simulink model "gm_inc_enc_v26_vnl"  (R2022b)
settings: Solver=FixedStepDiscrete  StartTime=0.0  StopTime=SimulationsDauer  RelTol=1e-3
undefined symbols (not defined in the file or in its folder): CW_CCW_Switch, d_axis_hit_CompareValue, DiscIntNeverNeededParam, f_ISR, IncPerTurn, inital_zero_speed_timeout, n_max, Offset_Position_elec, Offset_Position_mech, OmegaPerOverSampl, Periode, Phase_Delay_A, Phase_Delay_B, PolePair, QuadratureFactor, reciprocal_iterations, T_fpga, T_mech
libraries: simulink x25, hdlsllib x11, hdlmdlgenlib x4, dspsrcs4 x3, dspswit3 x2, spsEdgeDetectorLib x2, simulink_extras x1
(part 1 of 5)
settings Model: Creator=Wendel_ELSYS  LastModifiedBy=Admin
settings SolverCC: ConcurrentTasks=on  AlgebraicLoopSolver=TrustRegion  MinimalZcImpactIntegration=on
settings DataIOCC: LimitDataPoints=on  SaveFormat=Array
settings OptimizationCC: BlockReduction=off  ConditionallyExecuteInputs=off  DefaultParameterBehavior=Inlined  InheritOutputTypeSmallerThanSingle=on  LifeSpan=inf
settings DebuggingCC: ReadBeforeWriteMsg=DisableAll  WriteAfterWriteMsg=DisableAll  WriteAfterReadMsg=DisableAll  AlgebraicLoopMsg=error  InheritedTsInSrcMsg=none  SingleTaskRateTransMsg=error  ParameterOverflowMsg=none  UnconnectedInputMsg=warning  UnconnectedOutputMsg=warning  UnconnectedLineMsg=warning  SFUnexpectedBacktrackingDiag=warning  SFNoUnconditionalDefaultTransitionDiag=warning  SFExecutionAtInitializationDiag=none  SFMachineParentedDataDiag=warning  ArithmeticOperatorsInVariantConditions=warning
settings HardwareCC: ProdBitPerPointer=32  ProdBitPerSizeT=32  ProdBitPerPtrDiffT=32  ProdLargestAtomicFloat=None  ProdIntDivRoundTo=Undefined  ProdEndianess=Unspecified  ProdWordSize=32  ProdHWDeviceType=ASIC/FPGA->ASIC/FPGA  ProdEqTarget=off
settings ModelReferenceCC: UpdateModelReferenceTargets=IfOutOfDate  EnableRefExpFcnMdlSchedulingChecks=on  PropagateSignalLabelsOutOfModel=off
settings SFSimCC: SFSimEcho=off  SimUseLocalCustomCode=off  CustomCodeUndefinedFunction=UseInterfaceOnly
settings RTWCC: RTWUseLocalCustomCode=off  DLArmComputeVersion=19.05
settings CodeAppCC: StateflowObjectComments=on
settings GRTTargetCC: TargetLangStandard=C89/C90 (ANSI)
settings ConfigComp: CovMetricSettings=dw  CovSaveCumulativeToWorkspaceVar=on  CovSaveSingleToWorkspaceVar=on  CovExternalEMLEnable=off
settings SimscapeCC: SimscapeNormalizeSystem=off

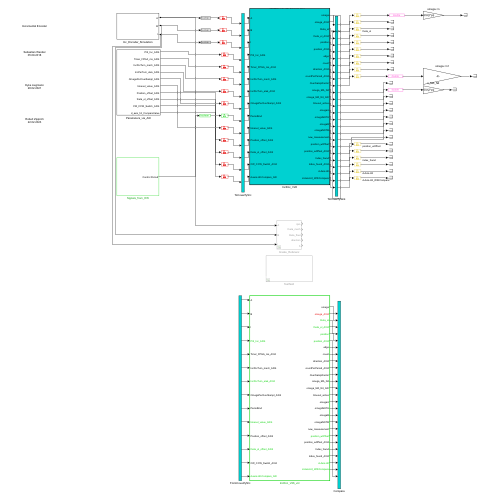
[thumbnail: Simulink's stored preview of the top-level diagram]
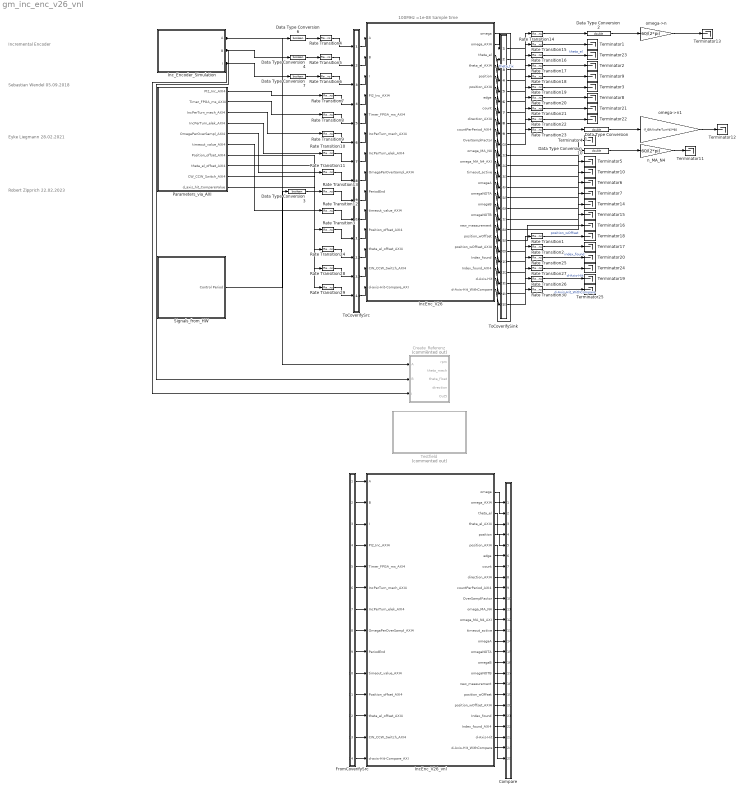
== system gm_inc_enc_v26_vnl ==
  note: 100MHz =1e-08 Sample time
  note: Sebastian Wendel
      | 05.09.2018
  note: Incremental Encoder
  note: Eyke Liegmann
      | 28.02.2021
  note: Robert Zipprich
      | 22.02.2023
  Compare : Subsystem
      mask Display: disp('')
  Create_Referenz : Subsystem  Commented=on
  Data Type Conversion1 : DataTypeConversion  OutDataTypeStr=double  SaturateOnIntegerOverflow=off  RndMeth=Floor
  Data Type Conversion10 : DataTypeConversion  OutDataTypeStr=double  SaturateOnIntegerOverflow=off  RndMeth=Floor
  Data Type Conversion2 : DataTypeConversion  OutDataTypeStr=double  SaturateOnIntegerOverflow=off  RndMeth=Floor
  Data Type Conversion{3..4,6..7} (4 alike) : DataTypeConversion  OutDataTypeStr=boolean  SaturateOnIntegerOverflow=off  RndMeth=Floor
  FromCoverifySrc : Subsystem
      mask Display: disp('')
  IncEnc_V26 : Subsystem  TreatAsAtomicUnit=on
  IncEnc_V26_vnl : Subsystem  TreatAsAtomicUnit=on
  Inc_Encoder_Simulation : Subsystem
  Parameters_via_AXI : Subsystem
  Rate Transition{1..2,14..23,25..27,30} (16 alike) : RateTransition  Deterministic=off  OutPortSampleTime=T_mech
  Rate Transition{3..13,24,28..29} (14 alike) : RateTransition  Deterministic=off  OutPortSampleTime=T_fpga
  Signals_from_HW : Subsystem
  Terminator{1..25} (25 alike) : Terminator
  Testfield : Subsystem  Commented=on
  ToCoverifySink : Subsystem
      mask Display: disp('')
  ToCoverifySrc : Subsystem
      mask Display: disp('')
  n_MA_N4 : Gain  Gain=60/(2*pi)  OutDataTypeStr=double
  omega->n : Gain  Gain=60/(2*pi)  OutDataTypeStr=double
  omega->n1 : Gain  Gain=(f_ISR/(IncPerTurn*4))*60  OutDataTypeStr=double
  wires:
  Data Type Conversion6/1 -> Rate Transition4/1
  Data Type Conversion4/1 -> Rate Transition5/1
  Data Type Conversion7/1 -> Rate Transition6/1
  omega->n/1 -> Terminator13/1
  Data Type Conversion2/1 -> omega->n/1
  Data Type Conversion1/1 -> omega->n1/1
  Data Type Conversion3/1 -> Rate Transition13/1
  Rate Transition14/1 -> Data Type Conversion2/1
  Rate Transition15/1 -> Terminator1/1
  Rate Transition17/1 -> Terminator2/1
  Rate Transition19/1 -> Terminator3/1
  Rate Transition23/1 -> Data Type Conversion1/1
  Data Type Conversion10/1 -> n_MA_N4/1
  Rate Transition20/1 -> Terminator8/1
  Rate Transition18/1 -> Terminator9/1
  n_MA_N4/1 -> Terminator11/1
  omega->n1/1 -> Terminator12/1
  Parameters_via_AXI/1(PI2_Inc_AXI4) -> Rate Transition7/1
  Parameters_via_AXI/2(Timer_FPGA_ms_AXI4) -> Rate Transition8/1
  Parameters_via_AXI/3(IncPerTurn_mech_AXI4) -> Rate Transition9/1
  Parameters_via_AXI/4(IncPerTurn_elek_AXI4) -> Rate Transition10/1
  Parameters_via_AXI/5(OmegaPerOverSampl_AXI4) -> Rate Transition11/1
  Parameters_via_AXI/6(timeout_value_AXI4) -> Rate Transition12/1
  Inc_Encoder_Simulation/2(B) -> Create_Referenz/2(B), Data Type Conversion4/1
  Inc_Encoder_Simulation/3(I) -> Create_Referenz/3(I), Data Type Conversion7/1
  Inc_Encoder_Simulation/1(A) -> Data Type Conversion6/1, Create_Referenz/1(A)
  Signals_from_HW/1(Control Period) -> Data Type Conversion3/1
  Rate Transition1/1 -> Terminator18/1  "position_wOffset"
  Rate Transition2/1 -> Terminator17/1
  Parameters_via_AXI/7(Position_offset_AXI4) -> Rate Transition3/1
  Parameters_via_AXI/8(theta_el_offset_AXI4) -> Rate Transition24/1
  Rate Transition25/1 -> Terminator20/1  "index_found"
  Rate Transition26/1 -> Terminator19/1  "d-Axis-Hit"
  Rate Transition22/1 -> Terminator22/1
  Rate Transition21/1 -> Terminator21/1
  Rate Transition16/1 -> Terminator23/1  "theta_el"
  Rate Transition27/1 -> Terminator24/1
  Parameters_via_AXI/9(CW_CCW_Switch_AXI4) -> Rate Transition28/1
  Parameters_via_AXI/10(d_axis_hit_CompareValue) -> Rate Transition29/1
  Rate Transition30/1 -> Terminator25/1  "d-Axis-Hit_WithCompare"
  ToCoverifySrc/1(out1) -> IncEnc_V26/1(A)
  ToCoverifySrc/2(out2) -> IncEnc_V26/2(B)
  ToCoverifySrc/3(out3) -> IncEnc_V26/3(I)
  ToCoverifySrc/4(out4) -> IncEnc_V26/4(PI2_Inc_AXI4)
  ToCoverifySrc/5(out5) -> IncEnc_V26/5(Timer_FPGA_ms_AXI4)
  ToCoverifySrc/6(out6) -> IncEnc_V26/6(IncPerTurn_mech_AXI4)
  ToCoverifySrc/7(out7) -> IncEnc_V26/7(IncPerTurn_elek_AXI4)
  ToCoverifySrc/8(out8) -> IncEnc_V26/8(OmegaPerOverSampl_AXI4)
  ToCoverifySrc/9(out9) -> IncEnc_V26/9(PeriodEnd)
  ToCoverifySrc/10(out10) -> IncEnc_V26/10(timeout_value_AXI4)
  ToCoverifySrc/11(out11) -> IncEnc_V26/11(Position_offset_AXI4)
  ToCoverifySrc/12(out12) -> IncEnc_V26/12(theta_el_offset_AXI4)
  ToCoverifySrc/13(out13) -> IncEnc_V26/13(CW_CCW_Switch_AXI4)
  ToCoverifySrc/14(out14) -> IncEnc_V26/14(d-axis-Hit-Compare_AXI)
  IncEnc_V26/1(omega) -> ToCoverifySink/1(in1)
  IncEnc_V26/2(omega_AXI4) -> ToCoverifySink/2(in2)
  IncEnc_V26/3(theta_el) -> ToCoverifySink/3(in3)  "theta_fix"
  IncEnc_V26/4(theta_el_AXI4) -> ToCoverifySink/4(in4)
  IncEnc_V26/5(position) -> ToCoverifySink/5(in5)
  IncEnc_V26/6(position_AXI4) -> ToCoverifySink/6(in6)
  IncEnc_V26/7(edge) -> ToCoverifySink/7(in7)
  IncEnc_V26/8(count) -> ToCoverifySink/8(in8)
  IncEnc_V26/9(direction_AXI4) -> ToCoverifySink/9(in9)
  IncEnc_V26/10(countPerPeriod_AXI4) -> ToCoverifySink/10(in10)
  IncEnc_V26/11(OverSamplFactor) -> ToCoverifySink/11(in11)
  IncEnc_V26/12(omega_MA_N4) -> ToCoverifySink/12(in12)
  IncEnc_V26/13(omega_MA_N4_AXI) -> ToCoverifySink/13(in13)
  IncEnc_V26/14(timeout_active) -> ToCoverifySink/14(in14)
  IncEnc_V26/15(omegaA) -> ToCoverifySink/15(in15)
  IncEnc_V26/16(omegaNOTA) -> ToCoverifySink/16(in16)
  IncEnc_V26/17(omegaB) -> ToCoverifySink/17(in17)
  IncEnc_V26/18(omegaNOTB) -> ToCoverifySink/18(in18)
  IncEnc_V26/19(new_measurement) -> ToCoverifySink/19(in19)
  IncEnc_V26/20(position_wOffset) -> ToCoverifySink/20(in20)
  IncEnc_V26/21(position_wOffset_AXI4) -> ToCoverifySink/21(in21)
  IncEnc_V26/22(Index_found) -> ToCoverifySink/22(in22)
  IncEnc_V26/23(Index_found_AXI4) -> ToCoverifySink/23(in23)
  IncEnc_V26/24(d-Axis-Hit) -> ToCoverifySink/24(in24)
  IncEnc_V26/25(d-Axis-Hit_WithCompare) -> ToCoverifySink/25(in25)
  Rate Transition4/1 -> ToCoverifySrc/1(in1)
  Rate Transition5/1 -> ToCoverifySrc/2(in2)
  Rate Transition6/1 -> ToCoverifySrc/3(in3)
  Rate Transition7/1 -> ToCoverifySrc/4(in4)
  Rate Transition8/1 -> ToCoverifySrc/5(in5)
  Rate Transition9/1 -> ToCoverifySrc/6(in6)
  Rate Transition10/1 -> ToCoverifySrc/7(in7)
  Rate Transition11/1 -> ToCoverifySrc/8(in8)
  Rate Transition13/1 -> ToCoverifySrc/9(in9)
  Rate Transition12/1 -> ToCoverifySrc/10(in10)
  Rate Transition3/1 -> ToCoverifySrc/11(in11)
  Rate Transition24/1 -> ToCoverifySrc/12(in12)
  Rate Transition28/1 -> ToCoverifySrc/13(in13)
  Rate Transition29/1 -> ToCoverifySrc/14(in14)
  ToCoverifySink/1(out1) -> Rate Transition14/1
  ToCoverifySink/2(out2) -> Rate Transition15/1
  ToCoverifySink/3(out3) -> Rate Transition16/1
  ToCoverifySink/4(out4) -> Rate Transition17/1
  ToCoverifySink/5(out5) -> Rate Transition18/1
  ToCoverifySink/6(out6) -> Rate Transition19/1
  ToCoverifySink/7(out7) -> Rate Transition20/1
  ToCoverifySink/8(out8) -> Rate Transition21/1
  ToCoverifySink/9(out9) -> Rate Transition22/1
  ToCoverifySink/10(out10) -> Rate Transition23/1
  ToCoverifySink/11(out11) -> Terminator4/1
  ToCoverifySink/12(out12) -> Data Type Conversion10/1
  ToCoverifySink/13(out13) -> Terminator5/1
  ToCoverifySink/14(out14) -> Terminator10/1
  ToCoverifySink/15(out15) -> Terminator6/1
  ToCoverifySink/16(out16) -> Terminator7/1
  ToCoverifySink/17(out17) -> Terminator14/1
  ToCoverifySink/18(out18) -> Terminator15/1
  ToCoverifySink/19(out19) -> Terminator16/1
  ToCoverifySink/20(out20) -> Rate Transition1/1
  ToCoverifySink/21(out21) -> Rate Transition2/1
  ToCoverifySink/22(out22) -> Rate Transition25/1
  ToCoverifySink/23(out23) -> Rate Transition27/1
  ToCoverifySink/24(out24) -> Rate Transition26/1
  ToCoverifySink/25(out25) -> Rate Transition30/1
  FromCoverifySrc/1(out1) -> IncEnc_V26_vnl/1(A)
  FromCoverifySrc/2(out2) -> IncEnc_V26_vnl/2(B)
  FromCoverifySrc/3(out3) -> IncEnc_V26_vnl/3(I)
  FromCoverifySrc/4(out4) -> IncEnc_V26_vnl/4(PI2_Inc_AXI4)
  FromCoverifySrc/5(out5) -> IncEnc_V26_vnl/5(Timer_FPGA_ms_AXI4)
  FromCoverifySrc/6(out6) -> IncEnc_V26_vnl/6(IncPerTurn_mech_AXI4)
  FromCoverifySrc/7(out7) -> IncEnc_V26_vnl/7(IncPerTurn_elek_AXI4)
  FromCoverifySrc/8(out8) -> IncEnc_V26_vnl/8(OmegaPerOverSampl_AXI4)
  FromCoverifySrc/9(out9) -> IncEnc_V26_vnl/9(PeriodEnd)
  FromCoverifySrc/10(out10) -> IncEnc_V26_vnl/10(timeout_value_AXI4)
  FromCoverifySrc/11(out11) -> IncEnc_V26_vnl/11(Position_offset_AXI4)
  FromCoverifySrc/12(out12) -> IncEnc_V26_vnl/12(theta_el_offset_AXI4)
  FromCoverifySrc/13(out13) -> IncEnc_V26_vnl/13(CW_CCW_Switch_AXI4)
  FromCoverifySrc/14(out14) -> IncEnc_V26_vnl/14(d-axis-Hit-Compare_AXI)
  IncEnc_V26_vnl/1(omega) -> Compare/1(in1)
  IncEnc_V26_vnl/2(omega_AXI4) -> Compare/2(in2)
  IncEnc_V26_vnl/3(theta_el) -> Compare/3(in3)
  IncEnc_V26_vnl/4(theta_el_AXI4) -> Compare/4(in4)
  IncEnc_V26_vnl/5(position) -> Compare/5(in5)
  IncEnc_V26_vnl/6(position_AXI4) -> Compare/6(in6)
  IncEnc_V26_vnl/7(edge) -> Compare/7(in7)
  IncEnc_V26_vnl/8(count) -> Compare/8(in8)
  IncEnc_V26_vnl/9(direction_AXI4) -> Compare/9(in9)
  IncEnc_V26_vnl/10(countPerPeriod_AXI4) -> Compare/10(in10)
  IncEnc_V26_vnl/11(OverSamplFactor) -> Compare/11(in11)
  IncEnc_V26_vnl/12(omega_MA_N4) -> Compare/12(in12)
  IncEnc_V26_vnl/13(omega_MA_N4_AXI) -> Compare/13(in13)
  IncEnc_V26_vnl/14(timeout_active) -> Compare/14(in14)
  IncEnc_V26_vnl/15(omegaA) -> Compare/15(in15)
  IncEnc_V26_vnl/16(omegaNOTA) -> Compare/16(in16)
  IncEnc_V26_vnl/17(omegaB) -> Compare/17(in17)
  IncEnc_V26_vnl/18(omegaNOTB) -> Compare/18(in18)
  IncEnc_V26_vnl/19(new_measurement) -> Compare/19(in19)
  IncEnc_V26_vnl/20(position_wOffset) -> Compare/20(in20)
  IncEnc_V26_vnl/21(position_wOffset_AXI4) -> Compare/21(in21)
  IncEnc_V26_vnl/22(Index_found) -> Compare/22(in22)
  IncEnc_V26_vnl/23(Index_found_AXI4) -> Compare/23(in23)
  IncEnc_V26_vnl/24(d-Axis-Hit) -> Compare/24(in24)
  IncEnc_V26_vnl/25(d-Axis-Hit_WithCompare) -> Compare/25(in25)

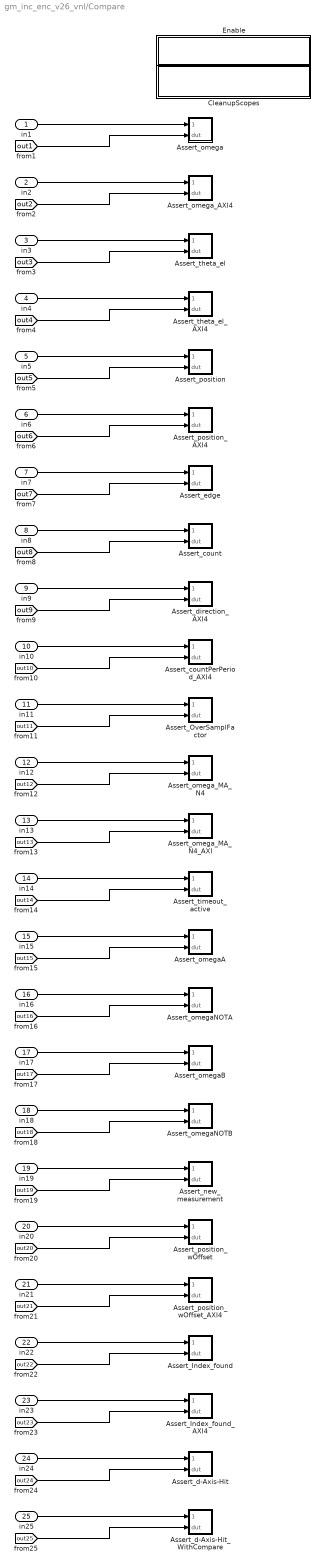
== system gm_inc_enc_v26_vnl/Compare ==
  in1 : Inport
  in2 : Inport  Port=2
  in3 : Inport  Port=3
  in4 : Inport  Port=4
  in5 : Inport  Port=5
  in6 : Inport  Port=6
  in7 : Inport  Port=7
  in8 : Inport  Port=8
  in9 : Inport  Port=9
  in10 : Inport  Port=10
  in11 : Inport  Port=11
  in12 : Inport  Port=12
  in13 : Inport  Port=13
  in14 : Inport  Port=14
  in15 : Inport  Port=15
  in16 : Inport  Port=16
  in17 : Inport  Port=17
  in18 : Inport  Port=18
  in19 : Inport  Port=19
  in20 : Inport  Port=20
  in21 : Inport  Port=21
  in22 : Inport  Port=22
  in23 : Inport  Port=23
  in24 : Inport  Port=24
  in25 : Inport  Port=25
  Assert_Index_found : Subsystem
      settings: LibrarySourceBlock=hdlmdlgenlib/AssertEq
  Assert_Index_found_AXI4 : Subsystem
      settings: LibrarySourceBlock=hdlmdlgenlib/AssertEq
  Assert_OverSamplFactor : Subsystem
      settings: LibrarySourceBlock=hdlmdlgenlib/AssertEq
  Assert_count : Subsystem
      settings: LibrarySourceBlock=hdlmdlgenlib/AssertEq
  Assert_countPerPeriod_AXI4 : Subsystem
      settings: LibrarySourceBlock=hdlmdlgenlib/AssertEq
  Assert_d-Axis-Hit : Subsystem
      settings: LibrarySourceBlock=hdlmdlgenlib/AssertEq
  Assert_d-Axis-Hit_WithCompare : Subsystem
      settings: LibrarySourceBlock=hdlmdlgenlib/AssertEq
  Assert_direction_AXI4 : Subsystem
      settings: LibrarySourceBlock=hdlmdlgenlib/AssertEq
  Assert_edge : Subsystem
      settings: LibrarySourceBlock=hdlmdlgenlib/AssertEq
  Assert_new_measurement : Subsystem
      settings: LibrarySourceBlock=hdlmdlgenlib/AssertEq
  Assert_omega : Subsystem
      settings: LibrarySourceBlock=hdlmdlgenlib/AssertEq
  Assert_omegaA : Subsystem
      settings: LibrarySourceBlock=hdlmdlgenlib/AssertEq
  Assert_omegaB : Subsystem
      settings: LibrarySourceBlock=hdlmdlgenlib/AssertEq
  Assert_omegaNOTA : Subsystem
      settings: LibrarySourceBlock=hdlmdlgenlib/AssertEq
  Assert_omegaNOTB : Subsystem
      settings: LibrarySourceBlock=hdlmdlgenlib/AssertEq
  Assert_omega_AXI4 : Subsystem
      settings: LibrarySourceBlock=hdlmdlgenlib/AssertEq
  Assert_omega_MA_N4 : Subsystem
      settings: LibrarySourceBlock=hdlmdlgenlib/AssertEq
  Assert_omega_MA_N4_AXI : Subsystem
      settings: LibrarySourceBlock=hdlmdlgenlib/AssertEq
  Assert_position : Subsystem
      settings: LibrarySourceBlock=hdlmdlgenlib/AssertEq
  Assert_position_AXI4 : Subsystem
      settings: LibrarySourceBlock=hdlmdlgenlib/AssertEq
  Assert_position_wOffset : Subsystem
      settings: LibrarySourceBlock=hdlmdlgenlib/AssertEq
  Assert_position_wOffset_AXI4 : Subsystem
      settings: LibrarySourceBlock=hdlmdlgenlib/AssertEq
  Assert_theta_el : Subsystem
      settings: LibrarySourceBlock=hdlmdlgenlib/AssertEq
  Assert_theta_el_AXI4 : Subsystem
      settings: LibrarySourceBlock=hdlmdlgenlib/AssertEq
  Assert_timeout_active : Subsystem
      settings: LibrarySourceBlock=hdlmdlgenlib/AssertEq
  CleanupScopes : Subsystem
      settings: OpenFcn=|
      | blkName = gcb; %self block
      | idx = regexp(blkName, '/CleanupScopes$', 'once');
      | blkParent = blkName(1:idx-1);
      | blks=find_system(blkParent, 'LookUnderMasks', 'all','blocktype', 'Scope');
      | for itr = 1:length(blks)
      | 	 hScopeCfg = get_param(blks{itr},'ScopeConfiguration');
      | 	 hScopeCfg.Visible = ~ hScopeCfg.Visible;
      | end
      | drawnow;
      mask Display: fprintf(message('hdlcoder:cosim:vnl_dblclick').getString());
  Enable : Subsystem
      settings: OpenFcn=|
      | blkName = gcb;
      | idx = regexp(blkName, '/Enable$', 'once');
      | blkParent = blkName(1:idx-1);
      | blks=find_system(blkParent, 'LookUnderMasks', 'all','blocktype', 'Assertion');
      | e = get_param(blks{1}, 'Enabled');
      | if strcmp(e, 'on'), f= 'off';, else, f = 'on';, end
      | for ii=1:length(blks), set_param(blks{ii}, 'Enabled', f);, end
      | set_param(gcb, 'MaskDisplay',['fprintf(message(''hdlcoder:cosim:vnl_dblclick_assertions'',','''',upper(e),'''',').getString())']);
      mask Display: fprintf(message('hdlcoder:cosim:vnl_dblclick_assertions','OFF').getString());
  wires:
  in1/1 -> Assert_omega/1(cosim)
  [out1] -> Assert_omega/2(dut)
  in2/1 -> Assert_omega_AXI4/1(cosim)
  [out2] -> Assert_omega_AXI4/2(dut)
  in3/1 -> Assert_theta_el/1(cosim)
  [out3] -> Assert_theta_el/2(dut)
  in4/1 -> Assert_theta_el_AXI4/1(cosim)
  [out4] -> Assert_theta_el_AXI4/2(dut)
  in5/1 -> Assert_position/1(cosim)
  [out5] -> Assert_position/2(dut)
  in6/1 -> Assert_position_AXI4/1(cosim)
  [out6] -> Assert_position_AXI4/2(dut)
  in7/1 -> Assert_edge/1(cosim)
  [out7] -> Assert_edge/2(dut)
  in8/1 -> Assert_count/1(cosim)
  [out8] -> Assert_count/2(dut)
  in9/1 -> Assert_direction_AXI4/1(cosim)
  [out9] -> Assert_direction_AXI4/2(dut)
  in10/1 -> Assert_countPerPeriod_AXI4/1(cosim)
  [out10] -> Assert_countPerPeriod_AXI4/2(dut)
  in11/1 -> Assert_OverSamplFactor/1(cosim)
  [out11] -> Assert_OverSamplFactor/2(dut)
  in12/1 -> Assert_omega_MA_N4/1(cosim)
  [out12] -> Assert_omega_MA_N4/2(dut)
  in13/1 -> Assert_omega_MA_N4_AXI/1(cosim)
  [out13] -> Assert_omega_MA_N4_AXI/2(dut)
  in14/1 -> Assert_timeout_active/1(cosim)
  [out14] -> Assert_timeout_active/2(dut)
  in15/1 -> Assert_omegaA/1(cosim)
  [out15] -> Assert_omegaA/2(dut)
  in16/1 -> Assert_omegaNOTA/1(cosim)
  [out16] -> Assert_omegaNOTA/2(dut)
  in17/1 -> Assert_omegaB/1(cosim)
  [out17] -> Assert_omegaB/2(dut)
  in18/1 -> Assert_omegaNOTB/1(cosim)
  [out18] -> Assert_omegaNOTB/2(dut)
  in19/1 -> Assert_new_measurement/1(cosim)
  [out19] -> Assert_new_measurement/2(dut)
  in20/1 -> Assert_position_wOffset/1(cosim)
  [out20] -> Assert_position_wOffset/2(dut)
  in21/1 -> Assert_position_wOffset_AXI4/1(cosim)
  [out21] -> Assert_position_wOffset_AXI4/2(dut)
  in22/1 -> Assert_Index_found/1(cosim)
  [out22] -> Assert_Index_found/2(dut)
  in23/1 -> Assert_Index_found_AXI4/1(cosim)
  [out23] -> Assert_Index_found_AXI4/2(dut)
  in24/1 -> Assert_d-Axis-Hit/1(cosim)
  [out24] -> Assert_d-Axis-Hit/2(dut)
  in25/1 -> Assert_d-Axis-Hit_WithCompare/1(cosim)
  [out25] -> Assert_d-Axis-Hit_WithCompare/2(dut)

== system gm_inc_enc_v26_vnl/Create_Referenz ==
  note: Überprüfen der Ausgabe:
      | (1/((Wert in Periodfelt von Counter)*Inkremente))*60
      | z.B. (1/((2.5*0.000001)*5000))*60
  A : Inport
  B : Inport  Port=2
  I : Inport  Port=3
  HardwareTimer_FPGA_in_ms*InCrements1 : Constant  Value=T_mech*IncPerTurn  OutDataTypeStr=double  SampleTime=T_mech
  IncrementalEncoder_Floating : Subsystem  Commented=on
  "daQuadraturEncoder " : Gain  Commented=on  Gain=4
  n_aus_theta : Subsystem  Commented=on  TreatAsAtomicUnit=on
  poles : Constant  Value=PolePair  OutDataTypeStr=uint8  SampleTime=T_mech
  rpm : Outport
  theta_mech : Outport  Port=2
  theta_float : Outport  Port=3
  direction : Outport  Port=4
  Out5 : Outport  Port=5
  wires:
  n_aus_theta/1(rpm) -> "daQuadraturEncoder "/1
  A/1 -> IncrementalEncoder_Floating/1(A), n_aus_theta/1(count)
  B/1 -> IncrementalEncoder_Floating/2(B)
  IncrementalEncoder_Floating/3(theta_elec) -> theta_float/1  "theta_float"
  poles/1 -> IncrementalEncoder_Floating/4(poles)
  I/1 -> IncrementalEncoder_Floating/3(I)
  HardwareTimer_FPGA_in_ms*InCrements1/1 -> n_aus_theta/2(T)
  IncrementalEncoder_Floating/4(direction) -> direction/1
  IncrementalEncoder_Floating/1(rpm) -> rpm/1
  "daQuadraturEncoder "/1 -> Out5/1
  IncrementalEncoder_Floating/2(theta_mech) -> theta_mech/1

== system gm_inc_enc_v26_vnl/FromCoverifySrc ==
  out1 : Outport
  out2 : Outport  Port=2
  out3 : Outport  Port=3
  out4 : Outport  Port=4
  out5 : Outport  Port=5
  out6 : Outport  Port=6
  out7 : Outport  Port=7
  out8 : Outport  Port=8
  out9 : Outport  Port=9
  out10 : Outport  Port=10
  out11 : Outport  Port=11
  out12 : Outport  Port=12
  out13 : Outport  Port=13
  out14 : Outport  Port=14
  wires:
  [in1] -> out1/1
  [in2] -> out2/1
  [in3] -> out3/1
  [in4] -> out4/1
  [in5] -> out5/1
  [in6] -> out6/1
  [in7] -> out7/1
  [in8] -> out8/1
  [in9] -> out9/1
  [in10] -> out10/1
  [in11] -> out11/1
  [in12] -> out12/1
  [in13] -> out13/1
  [in14] -> out14/1

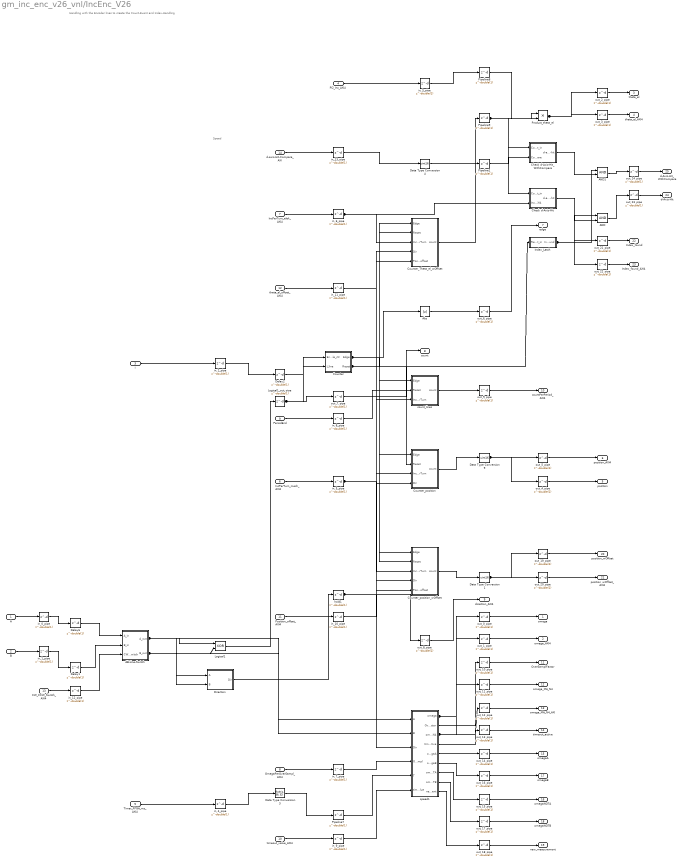
== system gm_inc_enc_v26_vnl/IncEnc_V26 ==
  note: Handling with the Encoder lines to create the Count-Event and Index-Handling
  note: Speed
  A : Inport  OutDataTypeStr=boolean  PortDimensions=1  SampleTime=1e-08
  B : Inport  Port=2  OutDataTypeStr=boolean  PortDimensions=1  SampleTime=1e-08
  I : Inport  Port=3  OutDataTypeStr=boolean  PortDimensions=1  SampleTime=1e-08
  PI2_Inc_AXI4 : Inport  Port=4  OutDataTypeStr=fixdt(0, 24, 24)  PortDimensions=1  SampleTime=1e-08
  Timer_FPGA_ms_AXI4 : Inport  Port=5  OutDataTypeStr=fixdt(0, 32, 32)  PortDimensions=1  SampleTime=1e-08
  IncPerTurn_mech_AXI4 : Inport  Port=6  OutDataTypeStr=uint16  PortDimensions=1  SampleTime=1e-08
  IncPerTurn_elek_AXI4 : Inport  Port=7  OutDataTypeStr=uint16  PortDimensions=1  SampleTime=1e-08
  OmegaPerOverSampl_AXI4 : Inport  Port=8  OutDataTypeStr=fixdt(1, 24, 11)  PortDimensions=1  SampleTime=1e-08
  PeriodEnd : Inport  Port=9  OutDataTypeStr=boolean  PortDimensions=1  SampleTime=1e-08
  timeout_value_AXI4 : Inport  Port=10  OutDataTypeStr=uint32  PortDimensions=1  SampleTime=1e-08
  Position_offset_AXI4 : Inport  Port=11  OutDataTypeStr=uint16  PortDimensions=1  SampleTime=1e-08
  theta_el_offset_AXI4 : Inport  Port=12  OutDataTypeStr=uint16  PortDimensions=1  SampleTime=1e-08
  CW_CCW_Switch_AXI4 : Inport  Port=13  OutDataTypeStr=boolean  PortDimensions=1  SampleTime=1e-08
  d-axis-Hit-Compare_AXI : Inport  Port=14  OutDataTypeStr=uint32  PortDimensions=1  SampleTime=1e-08
  AB-Line-Switch : Subsystem
  AND : Logic  AllPortsSameDT=off  OutDataTypeStr=boolean  SampleTime=1e-08
  AND1 : Logic  AllPortsSameDT=off  OutDataTypeStr=boolean  SampleTime=1e-08
  Abs : Abs  SampleTime=1e-08  OutDataTypeStr=fixdt(0, 1, 0)  RndMeth=Simplest  SaturateOnIntegerOverflow=off
  Check d-Axis-Hit : Subsystem
  Check d-Axis-Hit_WithCompare : Subsystem
  Counter : Subsystem
  Counter_Theta_el_wOffset : Subsystem
  Counter_position : Subsystem
  Counter_position_wOffset : Subsystem
  Data Type Conversion1 : DataTypeConversion  OutDataTypeStr=uint16  SampleTime=1e-08  SaturateOnIntegerOverflow=off  RndMeth=Floor
  Data Type Conversion3 : DataTypeConversion  OutDataTypeStr=fixdt(1, 38, 32)  SampleTime=1e-08  SaturateOnIntegerOverflow=off  RndMeth=Floor
  Data Type Conversion4 : DataTypeConversion  OutDataTypeStr=uint16  SampleTime=1e-08  SaturateOnIntegerOverflow=off  RndMeth=Floor
  Data Type Conversion9 : DataTypeConversion  OutDataTypeStr=uint16  SampleTime=1e-08  SaturateOnIntegerOverflow=off  RndMeth=Floor
  Delay1 : Delay  DelayLength=double(1)  InitialCondition=0  SampleTime=1e-08
  Delay2 : Delay  DelayLength=double(1)  InitialCondition=0  SampleTime=1e-08
  Delay6 : Delay  DelayLength=double(1)  InitialCondition=0  SampleTime=1e-08
  Direction : Subsystem
  Index_Latch : Subsystem
  Logical1 : Logic  Operator=XOR  AllPortsSameDT=off  OutDataTypeStr=boolean  SampleTime=1e-08
  Logical1_out_pipe : Delay  DelayLength=double(1)  InitialCondition=0  SampleTime=1e-08
  Pipeline{1,7..9} (4 alike) : Delay  DelayLength=double(1)  InitialCondition=0  SampleTime=1e-08
  Product_theta_el : Product  Inputs=**  OutDataTypeStr=fixdt(1, 24, 20)  SampleTime=1e-08
  count_lines : Subsystem
  hold1 : Delay  DelayLength=double(1)  InitialCondition=0  SampleTime=1e-08
  in_0_pipe : Delay  DelayLength=double(1)  InitialCondition=0  SampleTime=1e-08
  in_10_pipe : Delay  DelayLength=double(1)  InitialCondition=0  SampleTime=1e-08
  in_11_pipe : Delay  DelayLength=double(1)  InitialCondition=0  SampleTime=1e-08
  in_12_pipe : Delay  DelayLength=double(1)  InitialCondition=0  SampleTime=1e-08
  in_13_pipe : Delay  DelayLength=double(1)  InitialCondition=0  SampleTime=1e-08
  in_1_pipe : Delay  DelayLength=double(1)  InitialCondition=0  SampleTime=1e-08
  in_2_pipe : Delay  DelayLength=double(1)  InitialCondition=0  SampleTime=1e-08
  in_3_pipe : Delay  DelayLength=double(1)  InitialCondition=0  SampleTime=1e-08
  in_4_pipe : Delay  DelayLength=double(1)  InitialCondition=0  SampleTime=1e-08
  in_5_pipe : Delay  DelayLength=double(1)  InitialCondition=0  SampleTime=1e-08
  in_6_pipe : Delay  DelayLength=double(1)  InitialCondition=0  SampleTime=1e-08
  in_7_pipe : Delay  DelayLength=double(1)  InitialCondition=0  SampleTime=1e-08
  in_8_pipe : Delay  DelayLength=double(1)  InitialCondition=0  SampleTime=1e-08
  in_9_pipe : Delay  DelayLength=double(1)  InitialCondition=0  SampleTime=1e-08
  out_0_pipe : Delay  DelayLength=double(1)  InitialCondition=0  SampleTime=1e-08
  out_10_pipe : Delay  DelayLength=double(1)  InitialCondition=0  SampleTime=1e-08
  out_11_pipe : Delay  DelayLength=double(1)  InitialCondition=0  SampleTime=1e-08
  out_12_pipe : Delay  DelayLength=double(1)  InitialCondition=0  SampleTime=1e-08
  out_13_pipe : Delay  DelayLength=double(1)  InitialCondition=0  SampleTime=1e-08
  out_14_pipe : Delay  DelayLength=double(1)  InitialCondition=0  SampleTime=1e-08
  out_15_pipe : Delay  DelayLength=double(1)  InitialCondition=0  SampleTime=1e-08
  out_16_pipe : Delay  DelayLength=double(1)  InitialCondition=0  SampleTime=1e-08
  out_17_pipe : Delay  DelayLength=double(1)  InitialCondition=0  SampleTime=1e-08
  out_18_pipe : Delay  DelayLength=double(1)  InitialCondition=0  SampleTime=1e-08
  out_19_pipe : Delay  DelayLength=double(1)  InitialCondition=0  SampleTime=1e-08
  out_1_pipe : Delay  DelayLength=double(1)  InitialCondition=0  SampleTime=1e-08
  out_20_pipe : Delay  DelayLength=double(1)  InitialCondition=0  SampleTime=1e-08
  out_21_pipe : Delay  DelayLength=double(1)  InitialCondition=0  SampleTime=1e-08
  out_22_pipe : Delay  DelayLength=double(1)  InitialCondition=0  SampleTime=1e-08
  out_23_pipe : Delay  DelayLength=double(1)  InitialCondition=0  SampleTime=1e-08
  out_24_pipe : Delay  DelayLength=double(1)  InitialCondition=0  SampleTime=1e-08
  out_2_pipe : Delay  DelayLength=double(1)  InitialCondition=0  SampleTime=1e-08
  out_3_pipe : Delay  DelayLength=double(1)  InitialCondition=0  SampleTime=1e-08
  out_4_pipe : Delay  DelayLength=double(1)  InitialCondition=0  SampleTime=1e-08
  out_5_pipe : Delay  DelayLength=double(1)  InitialCondition=0  SampleTime=1e-08
  out_6_pipe : Delay  DelayLength=double(1)  InitialCondition=0  SampleTime=1e-08
  out_7_pipe : Delay  DelayLength=double(1)  InitialCondition=0  SampleTime=1e-08
  out_8_pipe : Delay  DelayLength=double(1)  InitialCondition=0  SampleTime=1e-08
  out_9_pipe : Delay  DelayLength=double(1)  InitialCondition=0  SampleTime=1e-08
  speed1 : Subsystem
  omega : Outport  SampleTime=1e-08  VectorParamsAs1DForOutWhenUnconnected=off
  omega_AXI4 : Outport  Port=2  SampleTime=1e-08  VectorParamsAs1DForOutWhenUnconnected=off
  theta_el : Outport  Port=3  SampleTime=1e-08  VectorParamsAs1DForOutWhenUnconnected=off
  theta_el_AXI4 : Outport  Port=4  SampleTime=1e-08  VectorParamsAs1DForOutWhenUnconnected=off
  position : Outport  Port=5  SampleTime=1e-08  VectorParamsAs1DForOutWhenUnconnected=off
  position_AXI4 : Outport  Port=6  SampleTime=1e-08  VectorParamsAs1DForOutWhenUnconnected=off
  edge : Outport  Port=7  SampleTime=1e-08  VectorParamsAs1DForOutWhenUnconnected=off
  count : Outport  Port=8  SampleTime=1e-08  VectorParamsAs1DForOutWhenUnconnected=off
  direction_AXI4 : Outport  Port=9  SampleTime=1e-08  VectorParamsAs1DForOutWhenUnconnected=off
  countPerPeriod_AXI4 : Outport  Port=10  SampleTime=1e-08  VectorParamsAs1DForOutWhenUnconnected=off
  OverSamplFactor : Outport  Port=11  SampleTime=1e-08  VectorParamsAs1DForOutWhenUnconnected=off
  omega_MA_N4 : Outport  Port=12  SampleTime=1e-08  VectorParamsAs1DForOutWhenUnconnected=off
  omega_MA_N4_AXI : Outport  Port=13  SampleTime=1e-08  VectorParamsAs1DForOutWhenUnconnected=off
  timeout_active : Outport  Port=14  OutDataTypeStr=boolean  SampleTime=1e-08  VectorParamsAs1DForOutWhenUnconnected=off
  omegaA : Outport  Port=15  SampleTime=1e-08  VectorParamsAs1DForOutWhenUnconnected=off
  omegaNOTA : Outport  Port=16  SampleTime=1e-08  VectorParamsAs1DForOutWhenUnconnected=off
  omegaB : Outport  Port=17  SampleTime=1e-08  VectorParamsAs1DForOutWhenUnconnected=off
  omegaNOTB : Outport  Port=18  SampleTime=1e-08  VectorParamsAs1DForOutWhenUnconnected=off
  new_measurement : Outport  Port=19  OutDataTypeStr=boolean  SampleTime=1e-08  VectorParamsAs1DForOutWhenUnconnected=off
  position_wOffset : Outport  Port=20  SampleTime=1e-08  VectorParamsAs1DForOutWhenUnconnected=off
  position_wOffset_AXI4 : Outport  Port=21  SampleTime=1e-08  VectorParamsAs1DForOutWhenUnconnected=off
  Index_found : Outport  Port=22  SampleTime=1e-08  VectorParamsAs1DForOutWhenUnconnected=off
  Index_found_AXI4 : Outport  Port=23  SampleTime=1e-08  VectorParamsAs1DForOutWhenUnconnected=off
  d-Axis-Hit : Outport  Port=24  SampleTime=1e-08  VectorParamsAs1DForOutWhenUnconnected=off
  d-Axis-Hit_WithCompare : Outport  Port=25  SampleTime=1e-08  VectorParamsAs1DForOutWhenUnconnected=off
  wires:
  d-axis-Hit-Compare_AXI/1 -> in_13_pipe/1
  CW_CCW_Switch_AXI4/1 -> in_12_pipe/1
  theta_el_offset_AXI4/1 -> in_11_pipe/1
  Position_offset_AXI4/1 -> in_10_pipe/1
  timeout_value_AXI4/1 -> in_9_pipe/1
  PeriodEnd/1 -> in_8_pipe/1
  OmegaPerOverSampl_AXI4/1 -> in_7_pipe/1
  IncPerTurn_elek_AXI4/1 -> in_6_pipe/1
  IncPerTurn_mech_AXI4/1 -> in_5_pipe/1
  Timer_FPGA_ms_AXI4/1 -> in_4_pipe/1
  PI2_Inc_AXI4/1 -> in_3_pipe/1
  I/1 -> in_2_pipe/1
  B/1 -> in_1_pipe/1
  A/1 -> in_0_pipe/1
  Logical1/1 -> Logical1_out_pipe/1
  out_24_pipe/1 -> d-Axis-Hit_WithCompare/1
  out_23_pipe/1 -> d-Axis-Hit/1
  out_22_pipe/1 -> Index_found_AXI4/1
  out_21_pipe/1 -> Index_found/1
  out_20_pipe/1 -> position_wOffset_AXI4/1
  out_19_pipe/1 -> position_wOffset/1
  out_18_pipe/1 -> new_measurement/1
  out_17_pipe/1 -> omegaNOTB/1
  out_16_pipe/1 -> omegaB/1
  out_15_pipe/1 -> omegaNOTA/1
  out_14_pipe/1 -> omegaA/1
  out_13_pipe/1 -> timeout_active/1
  out_12_pipe/1 -> omega_MA_N4_AXI/1
  out_11_pipe/1 -> omega_MA_N4/1
  out_10_pipe/1 -> OverSamplFactor/1
  out_9_pipe/1 -> countPerPeriod_AXI4/1
  out_8_pipe/1 -> direction_AXI4/1
  out_7_pipe/1 -> count/1
  out_6_pipe/1 -> edge/1
  out_5_pipe/1 -> position_AXI4/1
  out_4_pipe/1 -> position/1
  out_3_pipe/1 -> theta_el_AXI4/1
  out_2_pipe/1 -> theta_el/1
  out_1_pipe/1 -> omega_AXI4/1
  out_0_pipe/1 -> omega/1
  speed1/9(new_measurement) -> out_18_pipe/1
  speed1/8(omegaNOTB) -> out_17_pipe/1
  speed1/7(omegaNOTA) -> out_15_pipe/1
  speed1/6(omegaB) -> out_16_pipe/1
  speed1/5(omegaA) -> out_14_pipe/1
  speed1/4(timeout_active) -> out_13_pipe/1
  speed1/3(omega_MA_N4) -> out_11_pipe/1, out_12_pipe/1
  speed1/2(OverSamplFactor) -> out_10_pipe/1
  speed1/1(omega) -> out_0_pipe/1, out_1_pipe/1
  hold1/1 -> Counter_position_wOffset/4(Dir), Counter_Theta_el_wOffset/4(Dir), Counter_position/4(Dir), speed1/3(Dir), out_8_pipe/1
  count_lines/1(count) -> out_9_pipe/1
  Product_theta_el/1 -> out_2_pipe/1, out_3_pipe/1
  Pipeline9/1 -> Check d-Axis-Hit/1(Count_in), Check d-Axis-Hit_WithCompare/1(Count_in), Product_theta_el/1
  Pipeline8/1 -> Product_theta_el/2
  Pipeline7/1 -> speed1/5(T)
  Pipeline1/1 -> Check d-Axis-Hit_WithCompare/2(Counter_Compare)
  Logical1_out_pipe/1 -> Counter/1(Enable_ctr), out_7_pipe/1
  Index_Latch/1(Index_found) -> out_21_pipe/1, out_22_pipe/1, AND/1, AND1/1
  Direction/1(Dir) -> hold1/1
  Delay6/1 -> AB-Line-Switch/1(A_in)
  Delay2/1 -> Counter/2(I_line)
  Delay1/1 -> AB-Line-Switch/2(B_in)
  Data Type Conversion9/1 -> out_4_pipe/1, out_5_pipe/1
  Data Type Conversion4/1 -> Pipeline1/1
  Data Type Conversion3/1 -> Pipeline7/1
  Data Type Conversion1/1 -> out_19_pipe/1, out_20_pipe/1
  Counter_position_wOffset/1(count) -> Data Type Conversion1/1
  Counter_position/1(count) -> Data Type Conversion9/1
  Counter_Theta_el_wOffset/1(count) -> Pipeline9/1
  Counter/2(Reset) -> Index_Latch/1(Reset_in), Counter_position_wOffset/2(Reset), Counter_Theta_el_wOffset/2(Reset), Counter_position/2(Reset)
  Counter/1(Edge) -> count_lines/1(Edge), Counter_position_wOffset/1(Edge), Counter_Theta_el_wOffset/1(Edge), Counter_position/1(Edge), Abs/1
  Check d-Axis-Hit_WithCompare/1(d-axis-hit) -> AND1/2
  Check d-Axis-Hit/1(d-axis-hit) -> AND/2
  Abs/1 -> out_6_pipe/1
  AND1/1 -> out_24_pipe/1
  AND/1 -> out_23_pipe/1
  AB-Line-Switch/2(B_out) -> Direction/2(B), speed1/2(B), Logical1/2
  AB-Line-Switch/1(A_out) -> Direction/1(A), speed1/1(A), Logical1/1
  in_13_pipe/1 -> Data Type Conversion4/1
  in_12_pipe/1 -> AB-Line-Switch/3(CW_CCW_Switch)
  in_11_pipe/1 -> Counter_Theta_el_wOffset/5(Position_offset)
  in_10_pipe/1 -> Counter_position_wOffset/5(Position_offset)
  in_9_pipe/1 -> speed1/6(timeout_value)
  in_8_pipe/1 -> count_lines/2(Reset)
  in_7_pipe/1 -> speed1/4(OmegaPerOverSampl)
  in_6_pipe/1 -> Check d-Axis-Hit/2(IncPerTurn_elek_AXI4), Counter_Theta_el_wOffset/3(IncsPerTurn)
  in_5_pipe/1 -> count_lines/3(IncsPerTurn), Counter_position_wOffset/3(IncsPerTurn), Counter_position/3(IncsPerTurn)
  in_4_pipe/1 -> Data Type Conversion3/1
  in_3_pipe/1 -> Pipeline8/1
  in_2_pipe/1 -> Delay2/1
  in_1_pipe/1 -> Delay1/1
  in_0_pipe/1 -> Delay6/1

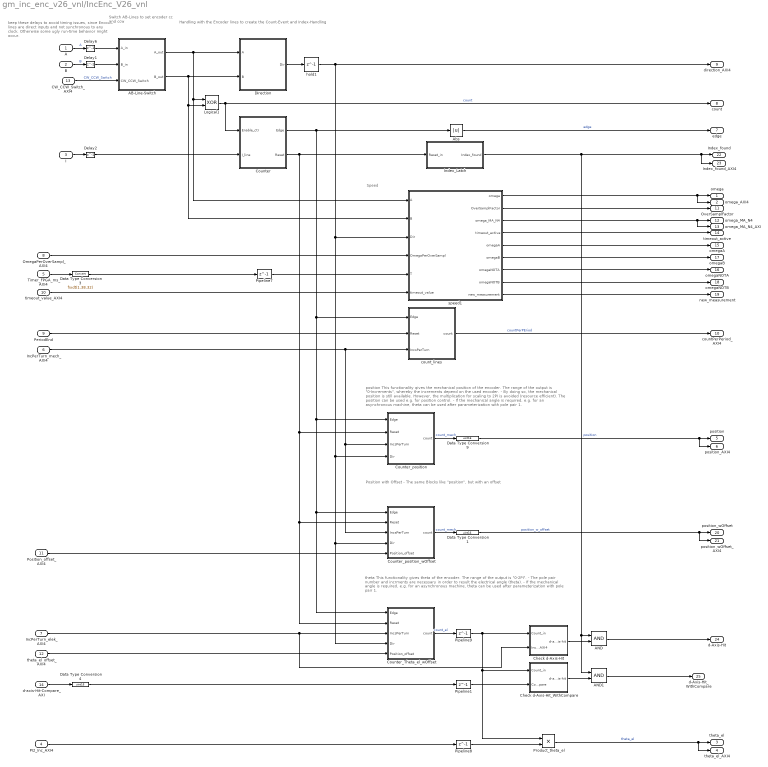
== system gm_inc_enc_v26_vnl/IncEnc_V26_vnl ==
  note: Position with Offset
      | - The same Blocks like "position", but with an offset
  note: keep these delays to avoid timing issues,
      | since Encoder lines are direct inputs and
      | not synchronous to any clock.
      | Otherwise some ugly run-time
      | behavior might occur.
  note: theta
      | This functionality gives theta of the encoder. The range of the output is "0-2PI".
      | - The pole pair number and incrments are necessary in order to result the electrical angle (theta).
      | - If the mechanical angle is required, e.g. for an asynchronous machine, theta can be used after parameterization with pole pair 1.
  note: position
      | This functionality gives the mechanical position of the encoder. The range of the output is "0-Increments", whereby the increments depend on the used encoder.
      | - By doing so, the mechanical position is still available. However, the multiplication for scaling to 2PI is avoided (resource efficient). The position can be used e.g. for position control.
      | - If the mechanical angle is required, e.g. for an asynchronous machine, theta can be used after parameterization with pole pair 1.
  note: Speed
  note: Handling with the Encoder lines to create the Count-Event and Index-Handling
  note: Switch AB-Lines to set
      | encoder cc and ccw
  A : Inport
  B : Inport  Port=2
  I : Inport  Port=3
  PI2_Inc_AXI4 : Inport  Port=4
  Timer_FPGA_ms_AXI4 : Inport  Port=5
  IncPerTurn_mech_AXI4 : Inport  Port=6
  IncPerTurn_elek_AXI4 : Inport  Port=7
  OmegaPerOverSampl_AXI4 : Inport  Port=8
  PeriodEnd : Inport  Port=9
  timeout_value_AXI4 : Inport  Port=10  OutDataTypeStr=uint32
  Position_offset_AXI4 : Inport  Port=11
  theta_el_offset_AXI4 : Inport  Port=12
  CW_CCW_Switch_AXI4 : Inport  Port=13
  d-axis-Hit-Compare_AXI : Inport  Port=14
  AB-Line-Switch : Subsystem
  AND : Logic  AllPortsSameDT=off  OutDataTypeStr=boolean
  AND1 : Logic  AllPortsSameDT=off  OutDataTypeStr=boolean
  Abs : Abs  OutDataTypeStr=fixdt(0,1,0)  RndMeth=Simplest  SaturateOnIntegerOverflow=off
  Check d-Axis-Hit : Subsystem
  Check d-Axis-Hit_WithCompare : Subsystem
  Counter : Subsystem  TreatAsAtomicUnit=on
  Counter_Theta_el_wOffset : Subsystem  TreatAsAtomicUnit=on
  Counter_position : Subsystem  TreatAsAtomicUnit=on
  Counter_position_wOffset : Subsystem  TreatAsAtomicUnit=on
  Data Type Conversion1 : DataTypeConversion  OutDataTypeStr=uint16  SaturateOnIntegerOverflow=off  RndMeth=Floor
  Data Type Conversion3 : DataTypeConversion  OutDataTypeStr=fixdt(1,38,32)  SaturateOnIntegerOverflow=off  RndMeth=Floor
  Data Type Conversion4 : DataTypeConversion  OutDataTypeStr=uint16  SaturateOnIntegerOverflow=off  RndMeth=Floor
  Data Type Conversion9 : DataTypeConversion  OutDataTypeStr=uint16  SaturateOnIntegerOverflow=off  RndMeth=Floor
  Delay1 : Delay  DelayLength=1  InitialCondition=0
  Delay2 : Delay  DelayLength=1  InitialCondition=0
  Delay6 : Delay  DelayLength=1  InitialCondition=0
  Direction : Subsystem  TreatAsAtomicUnit=on
  Index_Latch : Subsystem
  Logical1 : Logic  Operator=XOR  AllPortsSameDT=off  OutDataTypeStr=boolean
  Pipeline{1,7..9} (4 alike) : Delay  DelayLength=1
  Product_theta_el : Product  OutMin=[0]  OutMax=[2*pi]  OutDataTypeStr=fixdt(1,24,20)
  count_lines : Subsystem  TreatAsAtomicUnit=on
  hold1 : Delay  DelayLength=1
  speed1 : Subsystem
  omega : Outport  VectorParamsAs1DForOutWhenUnconnected=off
  omega_AXI4 : Outport  Port=2  VectorParamsAs1DForOutWhenUnconnected=off
  theta_el : Outport  Port=3  VectorParamsAs1DForOutWhenUnconnected=off
  theta_el_AXI4 : Outport  Port=4  VectorParamsAs1DForOutWhenUnconnected=off
  position : Outport  Port=5  VectorParamsAs1DForOutWhenUnconnected=off
  position_AXI4 : Outport  Port=6  VectorParamsAs1DForOutWhenUnconnected=off
  edge : Outport  Port=7  VectorParamsAs1DForOutWhenUnconnected=off
  count : Outport  Port=8  VectorParamsAs1DForOutWhenUnconnected=off
  direction_AXI4 : Outport  Port=9  VectorParamsAs1DForOutWhenUnconnected=off
  countPerPeriod_AXI4 : Outport  Port=10  VectorParamsAs1DForOutWhenUnconnected=off
  OverSamplFactor : Outport  Port=11  VectorParamsAs1DForOutWhenUnconnected=off
  omega_MA_N4 : Outport  Port=12  VectorParamsAs1DForOutWhenUnconnected=off
  omega_MA_N4_AXI : Outport  Port=13  VectorParamsAs1DForOutWhenUnconnected=off
  timeout_active : Outport  Port=14  OutDataTypeStr=boolean  VectorParamsAs1DForOutWhenUnconnected=off
  omegaA : Outport  Port=15  VectorParamsAs1DForOutWhenUnconnected=off
  omegaNOTA : Outport  Port=16  VectorParamsAs1DForOutWhenUnconnected=off
  omegaB : Outport  Port=17  VectorParamsAs1DForOutWhenUnconnected=off
  omegaNOTB : Outport  Port=18  VectorParamsAs1DForOutWhenUnconnected=off
  new_measurement : Outport  Port=19  OutDataTypeStr=boolean  VectorParamsAs1DForOutWhenUnconnected=off
  position_wOffset : Outport  Port=20  VectorParamsAs1DForOutWhenUnconnected=off
  position_wOffset_AXI4 : Outport  Port=21  VectorParamsAs1DForOutWhenUnconnected=off
  Index_found : Outport  Port=22  VectorParamsAs1DForOutWhenUnconnected=off
  Index_found_AXI4 : Outport  Port=23  VectorParamsAs1DForOutWhenUnconnected=off
  d-Axis-Hit : Outport  Port=24  VectorParamsAs1DForOutWhenUnconnected=off
  d-Axis-Hit_WithCompare : Outport  Port=25  VectorParamsAs1DForOutWhenUnconnected=off
  wires:
  Data Type Conversion4/1 -> Pipeline1/1
  PI2_Inc_AXI4/1 -> Pipeline8/1
  Pipeline1/1 -> Check d-Axis-Hit_WithCompare/2(Counter_Compare)
  d-axis-Hit-Compare_AXI/1 -> Data Type Conversion4/1
  AND1/1 -> d-Axis-Hit_WithCompare/1
  Check d-Axis-Hit_WithCompare/1(d-axis-hit) -> AND1/2
  CW_CCW_Switch_AXI4/1 -> AB-Line-Switch/3(CW_CCW_Switch)  "CW_CCW_Switch"
  Delay1/1 -> AB-Line-Switch/2(B_in)
  Delay6/1 -> AB-Line-Switch/1(A_in)
  Index_Latch/1(Index_found) -> AND/1, AND1/1, Index_found/1, Index_found_AXI4/1
  AND/1 -> d-Axis-Hit/1
  Check d-Axis-Hit/1(d-axis-hit) -> AND/2
  Pipeline8/1 -> Product_theta_el/2
  Pipeline9/1 -> Check d-Axis-Hit/1(Count_in), Product_theta_el/1, Check d-Axis-Hit_WithCompare/1(Count_in)
  theta_el_offset_AXI4/1 -> Counter_Theta_el_wOffset/5(Position_offset)
  Delay2/1 -> Counter/2(I_line)
  I/1 -> Delay2/1
  Position_offset_AXI4/1 -> Counter_position_wOffset/5(Position_offset)
  Data Type Conversion1/1 -> position_wOffset/1, position_wOffset_AXI4/1  "position_w_offset"
  Counter_position_wOffset/1(count) -> Data Type Conversion1/1  "count_mech"
  AB-Line-Switch/2(B_out) -> Direction/2(B), Logical1/2, speed1/2(B)
  AB-Line-Switch/1(A_out) -> Direction/1(A), Logical1/1, speed1/1(A)
  speed1/9(new_measurement) -> new_measurement/1
  speed1/8(omegaNOTB) -> omegaNOTB/1
  speed1/6(omegaB) -> omegaB/1
  speed1/7(omegaNOTA) -> omegaNOTA/1
  speed1/5(omegaA) -> omegaA/1
  timeout_value_AXI4/1 -> speed1/6(timeout_value)
  speed1/4(timeout_active) -> timeout_active/1
  speed1/3(omega_MA_N4) -> omega_MA_N4/1, omega_MA_N4_AXI/1
  speed1/2(OverSamplFactor) -> OverSamplFactor/1
  speed1/1(omega) -> omega/1, omega_AXI4/1
  Pipeline7/1 -> speed1/5(T)
  OmegaPerOverSampl_AXI4/1 -> speed1/4(OmegaPerOverSampl)
  Data Type Conversion3/1 -> Pipeline7/1
  Timer_FPGA_ms_AXI4/1 -> Data Type Conversion3/1
  IncPerTurn_mech_AXI4/1 -> count_lines/3(IncsPerTurn), Counter_position_wOffset/3(IncsPerTurn), Counter_position/3(IncsPerTurn)
  IncPerTurn_elek_AXI4/1 -> Check d-Axis-Hit/2(IncPerTurn_elek_AXI4), Counter_Theta_el_wOffset/3(IncsPerTurn)
  Abs/1 -> edge/1  "edge"
  count_lines/1(count) -> countPerPeriod_AXI4/1  "countPerPEriod"
  PeriodEnd/1 -> count_lines/2(Reset)
  Direction/1(Dir) -> hold1/1
  Counter/1(Edge) -> Abs/1, count_lines/1(Edge), Counter_position_wOffset/1(Edge), Counter_Theta_el_wOffset/1(Edge), Counter_position/1(Edge)
  Counter/2(Reset) -> Index_Latch/1(Reset_in), Counter_position_wOffset/2(Reset), Counter_Theta_el_wOffset/2(Reset), Counter_position/2(Reset)
  Product_theta_el/1 -> theta_el_AXI4/1, theta_el/1  "theta_el"
  Counter_Theta_el_wOffset/1(count) -> Pipeline9/1  "count_el"
  Logical1/1 -> count/1, Counter/1(Enable_ctr)  "count"
  Data Type Conversion9/1 -> position/1, position_AXI4/1  "position"
  Counter_position/1(count) -> Data Type Conversion9/1  "count_mech"
  hold1/1 -> Counter_position_wOffset/4(Dir), Counter_Theta_el_wOffset/4(Dir), Counter_position/4(Dir), speed1/3(Dir), direction_AXI4/1
  B/1 -> Delay1/1  "B"
  A/1 -> Delay6/1  "A"

== system gm_inc_enc_v26_vnl/Inc_Encoder_Simulation ==
  Logical Operator1 : Logic  Operator=XOR  AllPortsSameDT=off  OutDataTypeStr=boolean
  Manual Switch : ManualSwitch
  Manual Switch1 : ManualSwitch
  Manual Switch2 : ManualSwitch
  Pulse Generator1 0.1 : DiscretePulseGenerator  PulseType=Time based  Period=Periode  PulseWidth=50  PhaseDelay=Phase_Delay_B  SampleTime=T_mech  VectorParams1D=off
  Pulse Generator2 : DiscretePulseGenerator  PulseType=Time based  Period=Periode  PulseWidth=50  PhaseDelay=Phase_Delay_A  SampleTime=T_mech  VectorParams1D=off
  Rate Transition : RateTransition  Deterministic=off  OutPortSampleTime=T_mech
  Rate Transition2 : RateTransition  Deterministic=off  OutPortSampleTime=T_mech
  Signal From Workspace : dspsrcs4/Signal From Workspace  Commented=on  X=A_ila  Ts=T_mech  nsamps=1  OutputAfterFinalValue=Setting to zero  ignoreOrWarnInputAndFrameLengths=off  OutputFrames=off
  Signal From Workspace1 : dspsrcs4/Signal From Workspace  Commented=on  X=B_ila  Ts=T_mech  nsamps=1  OutputAfterFinalValue=Setting to zero  ignoreOrWarnInputAndFrameLengths=off  OutputFrames=off
  Signal From Workspace2 : dspsrcs4/Signal From Workspace  Commented=on  X=I_ila  Ts=T_mech  nsamps=1  OutputAfterFinalValue=Setting to zero  ignoreOrWarnInputAndFrameLengths=off  OutputFrames=off
  Simulate_I_Line : dspswit3/Counter  Direction=Up  CountEvent=Either edge  CounterSize=User defined  MaxCount=IncPerTurn*4  InitialCount=123  Output=Hit  HitValue=IncPerTurn*4  ResetInput=off  SamplesPerFrame=1  Ts=1  CntDtype=double  HitDtype=Boolean
  A : Outport
  B : Outport  Port=2
  I : Outport  Port=3
  wires:
  Pulse Generator2/1 -> Rate Transition/1  "A"
  Signal From Workspace1/1 -> Manual Switch1/2
  Logical Operator1/1 -> Simulate_I_Line/1
  Manual Switch1/1 -> B/1, Logical Operator1/2
  Signal From Workspace/1 -> Manual Switch/2
  Manual Switch/1 -> A/1, Logical Operator1/1
  Pulse Generator1 0.1/1 -> Rate Transition2/1  "B"
  Rate Transition/1 -> Manual Switch/1
  Rate Transition2/1 -> Manual Switch1/1
  Signal From Workspace2/1 -> Manual Switch2/2
  Simulate_I_Line/1 -> Manual Switch2/1
  Manual Switch2/1 -> I/1  "I"

== system gm_inc_enc_v26_vnl/Parameters_via_AXI ==
  CW_CCW_Switch_REG : Constant  Value=CW_CCW_Switch  OutDataTypeStr=boolean  SampleTime=T_mech
  CW_CCW_Switch_REG1 : Constant  Value=d_axis_hit_CompareValue  OutDataTypeStr=uint32  SampleTime=T_mech
  Constant : Constant  OutDataTypeStr=boolean
  Constant1 : Constant  Value=0  OutDataTypeStr=boolean
  "EncoderIncsPerTurn_elek_REG " : Constant  Value=(IncPerTurn*QuadratureFactor)/PolePair  OutDataTypeStr=fixdt(0,16,0)  SampleTime=T_mech
  EncoderIncsPerTurn_mech_REG : Constant  Value=IncPerTurn*QuadratureFactor  OutDataTypeStr=fixdt(0,16,0)  SampleTime=T_mech
  EncoderPI2_Inc_elek_REG : Constant  Value=(2*pi/(IncPerTurn*QuadratureFactor))*PolePair  OutDataTypeStr=fixdt(0,24,24)  SampleTime=T_mech
  Encoder_Time_REG HardwareTimer_FPGA_in_s*Increments and divide by 2PI for scaling to rad : Constant  Value=(T_fpga*IncPerTurn)/(2*pi)  OutDataTypeStr=fixdt(0,32,32)  SampleTime=T_mech
  Manual Switch : ManualSwitch  CurrentSetting=0
  Manual Switch1 : ManualSwitch  CurrentSetting=0
  OverSamplingFactorInverseREG : Constant  Value=OmegaPerOverSampl  OutDataTypeStr=fixdt(1,24,11)  SampleTime=T_mech
  Position_Offset_REG : Constant  Value=Offset_Position_mech  OutDataTypeStr=fixdt(0,16,0)  SampleTime=T_mech
  theta_el_Offset_REG : Constant  Value=Offset_Position_elec  OutDataTypeStr=fixdt(0,16,0)  SampleTime=T_mech
  zero_speed_timeout_REG : Constant  Value=inital_zero_speed_timeout  OutDataTypeStr=uint32  SampleTime=T_mech
  PI2_Inc_AXI4 : Outport
  Timer_FPGA_ms_AXI4 : Outport  Port=2
  IncPerTurn_mech_AXI4 : Outport  Port=3
  IncPerTurn_elek_AXI4 : Outport  Port=4
  OmegaPerOverSampl_AXI4 : Outport  Port=5
  timeout_value_AXI4 : Outport  Port=6
  Position_offset_AXI4 : Outport  Port=7
  theta_el_offset_AXI4 : Outport  Port=8
  CW_CCW_Switch_AXI4 : Outport  Port=9
  d_axis_hit_CompareValue : Outport  Port=10
  wires:
  "EncoderIncsPerTurn_elek_REG "/1 -> IncPerTurn_elek_AXI4/1
  Encoder_Time_REG HardwareTimer_FPGA_in_s*Increments and divide by 2PI for scaling to rad/1 -> Timer_FPGA_ms_AXI4/1
  zero_speed_timeout_REG/1 -> timeout_value_AXI4/1
  OverSamplingFactorInverseREG/1 -> OmegaPerOverSampl_AXI4/1
  EncoderPI2_Inc_elek_REG/1 -> PI2_Inc_AXI4/1
  EncoderIncsPerTurn_mech_REG/1 -> IncPerTurn_mech_AXI4/1
  Position_Offset_REG/1 -> Position_offset_AXI4/1
  theta_el_Offset_REG/1 -> theta_el_offset_AXI4/1
  Constant/1 -> Manual Switch/1
  Constant1/1 -> Manual Switch/2
  CW_CCW_Switch_REG/1 -> Manual Switch1/1
  Manual Switch/1 -> Manual Switch1/2
  Manual Switch1/1 -> CW_CCW_Switch_AXI4/1
  CW_CCW_Switch_REG1/1 -> d_axis_hit_CompareValue/1

== system gm_inc_enc_v26_vnl/Signals_from_HW ==
  uCTakt : DiscretePulseGenerator  PulseType=Time based  Period=1/f_ISR  PulseWidth=f_ISR*T_fpga *100  SampleTime=T_mech  VectorParams1D=off
  Control Period : Outport
  wires:
  uCTakt/1 -> Control Period/1  "Control Period"

== system gm_inc_enc_v26_vnl/Testfield ==
  Cast To Boolean1 : DataTypeConversion  OutDataTypeStr=boolean  SaturateOnIntegerOverflow=off  RndMeth=Floor
  Constant1 : Constant  Value=256*4
  Constant2 : Constant
  Constant3 : Constant  Value=512
  Counter_position_wOffset : Subsystem  TreatAsAtomicUnit=on
  Index_Latch : Subsystem
  Pulse Generator : DiscretePulseGenerator  Period=10  SampleTime=1/10e3
  Pulse Generator1 : DiscretePulseGenerator  Period=100000  PhaseDelay=42505  SampleTime=1/10e3
  Scope : Scope  NumInputPorts=3
  Scope1 : Scope  NumInputPorts=2
  wires:
  Constant1/1 -> Counter_position_wOffset/3(IncsPerTurn)
  Pulse Generator/1 -> Counter_position_wOffset/1(Edge), Scope/1
  Constant3/1 -> Counter_position_wOffset/5(Position_offset)
  Constant2/1 -> Counter_position_wOffset/4(Dir)
  Cast To Boolean1/1 -> Scope/2, Scope1/1, Index_Latch/1(Reset_in), Counter_position_wOffset/2(Reset)
  Pulse Generator1/1 -> Cast To Boolean1/1
  Counter_position_wOffset/1(count) -> Scope/3  "count_mech"
  Index_Latch/1(Index_found) -> Scope1/2
